simulink model "nasaBatterysim"  (R2019a)
settings: Solver=ode4  StartTime=0.0  StopTime=64  FixedStep=.01  RelTol=1e-3
settings Model: Creator=tdarrah  LastModifiedBy=tdarrah
settings DebuggingCC: ArithmeticOperatorsInVariantConditions=warning

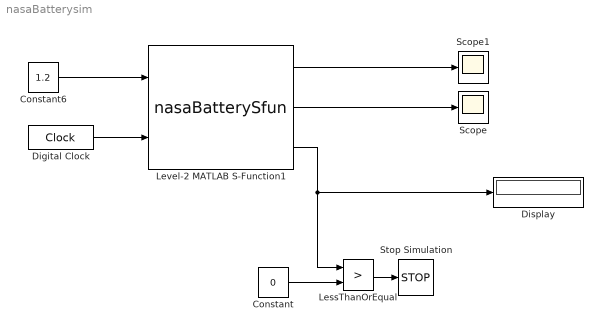
== system nasaBatterysim ==
  Constant : Constant  Value=0
  Constant6 : Constant  Value=1.2
  Digital Clock : DigitalClock
      mask Display: disp('simTime');
  Display : Display
  LessThanOrEqual : RelationalOperator  Operator=>  OutDataTypeStr=boolean  RndMeth=Simplest
  Level-2 MATLAB S-Function1 : M-S-Function  FunctionName=nasaBatterySfun  Parameters=batteryParams
      mask Display:
      | port_label('input', 1, 'current');
      | port_label('input', 2, 'simTime');
      | port_label('output', 1, 'voltage');
      | port_label('output', 2, 'soc');
      | port_label('output', 3, 'eod');
  Scope : Scope
  Scope1 : Scope
  Stop Simulation : Stop
  wires:
  Level-2 MATLAB S-Function1/3 -> Display/1, LessThanOrEqual/1
  Constant6/1 -> Level-2 MATLAB S-Function1/1
  Constant/1 -> LessThanOrEqual/2
  LessThanOrEqual/1 -> Stop Simulation/1
  Level-2 MATLAB S-Function1/2 -> Scope/1
  Level-2 MATLAB S-Function1/1 -> Scope1/1
  Digital Clock/1 -> Level-2 MATLAB S-Function1/2
